simulink model "sh1"  (R2014b)
settings: Solver=ode45  StartTime=0.0  StopTime=25.0  MaxStep=0.001  MinStep=0.0001  RelTol=1e-3
settings Model: Creator=Игорь  LastModifiedBy=Игорь

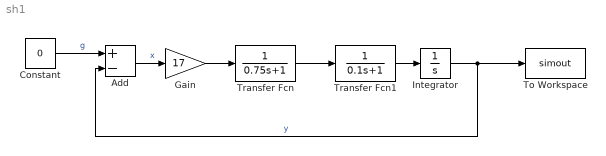
== system sh1 ==
  Add : Sum  Inputs=+-
  Constant : Constant  Value=0
  Gain : Gain  Gain=17
  Integrator : Integrator  InitialCondition=1
  To Workspace : ToWorkspace  VariableName=simout  SaveFormat=Timeseries  SampleTime=-1
  Transfer Fcn : TransferFcn  Denominator=[0.75 1]
  Transfer Fcn1 : TransferFcn  Denominator=[0.1 1]
  wires:
  Add/1 -> Gain/1  "x"
  Transfer Fcn1/1 -> Integrator/1
  Transfer Fcn/1 -> Transfer Fcn1/1
  Gain/1 -> Transfer Fcn/1
  Integrator/1 -> To Workspace/1, Add/2  "y"
  Constant/1 -> Add/1  "g"
